simulink model "Subsystem1"  (R2020b)
settings: Solver=VariableStepAuto  StartTime=0.0  StopTime=10  RelTol=1e-3
undefined symbols (not defined in the file or in its folder): Ki, kp
settings Model: Creator=intel  LastModifiedBy=intel
settings DataIOCC: SaveOutput=off  SaveTime=off

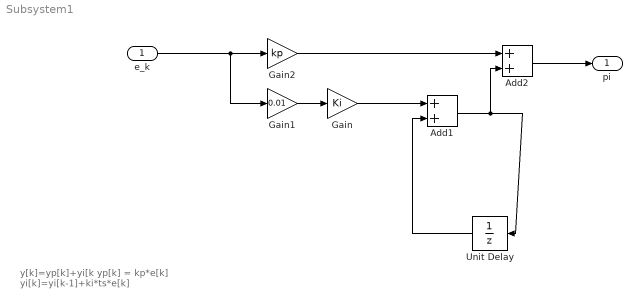
== system Subsystem1 ==
  note: y[k]=yp[k]+yi[k
      | yp[k] = kp*e[k]
      | yi[k]=yi[k-1]+ki*ts*e[k]
  e_k : Inport  OutDataTypeStr=double  PortDimensions=1  SampleTime=0
  Add1 : Sum
  Add2 : Sum
  Gain : Gain  Gain=Ki
  Gain1 : Gain  Gain=0.01
  Gain2 : Gain  Gain=kp
  Unit Delay : UnitDelay  SampleTime=-1  HasFrameUpgradeWarning=on
  pi : Outport  OutDataTypeStr=double  PortDimensions=1  SampleTime=0
  wires:
  Unit Delay/1 -> Add1/2
  Add1/1 -> Unit Delay/1, Add2/2
  Add2/1 -> pi/1
  Gain1/1 -> Gain/1
  Gain/1 -> Add1/1
  Gain2/1 -> Add2/1
  e_k/1 -> Gain2/1, Gain1/1
